simulink model "joint_test_dis_massless_2GBlks1"  (R2016b)
settings: Solver=VariableStepAuto  StartTime=0.0  StopTime=10.0  RelTol=1e-3
libraries: sm_lib x10
settings Model: Creator=smiller  LastModifiedBy=smiller

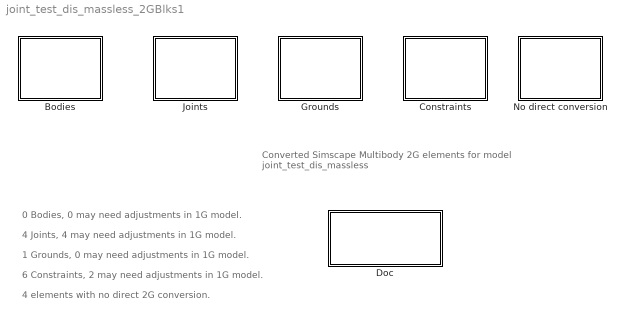
== system joint_test_dis_massless_2GBlks1 ==
  note: Converted Simscape Multibody 2G elements for model
      | joint_test_dis_massless
  note: 0 Bodies, 0 may need adjustments in 1G model.
  note: 4 Joints, 4 may need adjustments in 1G model.
  note: 1 Grounds, 0 may need adjustments in 1G model.
  note: 6 Constraints, 2 may need adjustments in 1G model.
  note: 4 elements with no direct 2G conversion.
  Bodies : Subsystem
  Constraints : Subsystem
  Doc : Subsystem
      settings: OpenFcn=web('SM1G2G_Warnings_Help.html');
      mask Display: disp('Double-click\nfor Information\nabout Diagnostics');
  Grounds : Subsystem
  Joints : Subsystem
  No direct conversion : Subsystem

== system joint_test_dis_massless_2GBlks1/Bodies ==

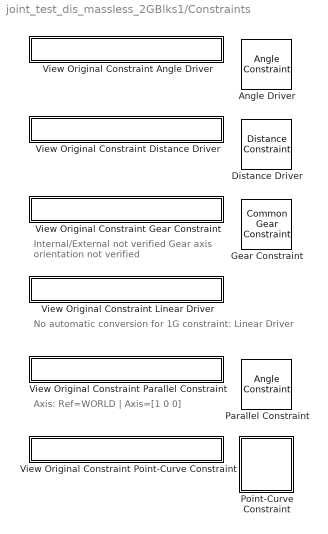
== system joint_test_dis_massless_2GBlks1/Constraints ==
  note: Internal/External not verified
      | Gear axis orientation not verified
  note: No automatic conversion for 1G constraint: Linear Driver
  note: Axis: Ref=WORLD | Axis=[1 0 0]
  Angle Driver : sm_lib/Constraints/Angle Constraint  ConstraintType=General  Angle=45  AngleUnits=deg  SenseSignedTorqueMagnitude=off  SenseTorque=off  SenseForce=off  WrenchDir=FollowerOnBase  WrenchFrame=BaseFrame
  Distance Driver : sm_lib/Constraints/Distance Constraint  Distance=1  DistanceUnits=m  SenseSignedForceMagnitude=off  SenseTorque=off  SenseForce=off  WrenchDir=FollowerOnBase  WrenchFrame=BaseFrame
  Gear Constraint : sm_lib/Gears and Couplings/Gears/Common Gear Constraint  GearType=External  SpecificationType=PitchCircleRadii  CenterDistance=20.0  CenterDistanceUnits=cm  GearRatio=1.0  BaseGearRadius=1  BaseGearRadiusUnits=m  FollGearRadius=1  FollGearRadiusUnits=m  AssemblyGearRotation=Free
  Parallel Constraint : sm_lib/Constraints/Angle Constraint  ConstraintType=Parallel  Angle=45  AngleUnits=deg  SenseSignedTorqueMagnitude=off  SenseTorque=off  SenseForce=off  WrenchDir=FollowerOnBase  WrenchFrame=BaseFrame
  Point-Curve Constraint : Subsystem
  View Original Constraint Angle Driver : Subsystem
      settings: OpenFcn=hilite_system('joint_test_dis_massless/Angle Driver');
      mask Display: disp(['View Original Constraint Angle Driver']);
  View Original Constraint Distance Driver : Subsystem
      settings: OpenFcn=hilite_system('joint_test_dis_massless/Distance Driver');
      mask Display: disp(['View Original Constraint Distance Driver']);
  View Original Constraint Gear Constraint : Subsystem
      settings: OpenFcn=hilite_system('joint_test_dis_massless/Gear Constraint');
      mask Display: disp(['View Original Constraint Gear Constraint']);
  View Original Constraint Linear Driver : Subsystem
      settings: OpenFcn=hilite_system('joint_test_dis_massless/Linear Driver');
      mask Display: disp(['View Original Constraint Linear Driver']);
  View Original Constraint Parallel Constraint : Subsystem
      settings: OpenFcn=hilite_system('joint_test_dis_massless/Parallel Constraint');
      mask Display: disp(['View Original Constraint Parallel Constraint']);
  View Original Constraint Point-Curve Constraint : Subsystem
      settings: OpenFcn=hilite_system('joint_test_dis_massless/Point-Curve Constraint');
      mask Display: disp(['View Original Constraint Point-Curve Constraint']);

== system joint_test_dis_massless_2GBlks1/Doc ==

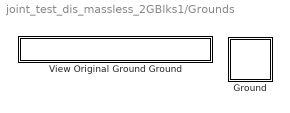
== system joint_test_dis_massless_2GBlks1/Grounds ==
  Ground : Subsystem
  View Original Ground Ground : Subsystem
      settings: OpenFcn=hilite_system('joint_test_dis_massless/Ground');
      mask Display: disp(['View Original Ground Ground']);

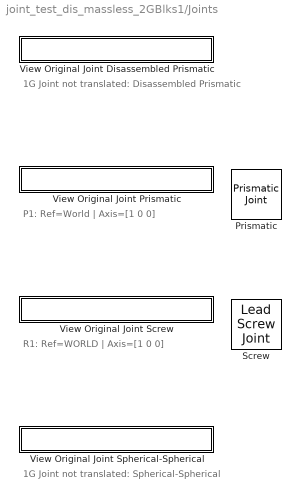
== system joint_test_dis_massless_2GBlks1/Joints ==
  note: 1G Joint not translated: Disassembled Prismatic
  note: P1: Ref=World | Axis=[1 0 0]
  note: R1: Ref=WORLD | Axis=[1 0 0]
  note: 1G Joint not translated: Spherical-Spherical
  Prismatic : sm_lib/Joints/Prismatic Joint  SenseConstraintForce=off  SenseConstraintForceX=off  SenseConstraintForceY=off  SenseConstraintForceZ=off  SenseConstraintTorque=off  SenseConstraintTorqueX=off  SenseConstraintTorqueY=off  SenseConstraintTorqueZ=off  SenseTotalForce=off  SenseTotalForceX=off  SenseTotalForceY=off  SenseTotalForceZ=off  SenseTotalTorque=off  SenseTotalTorqueX=off  SenseTotalTorqueY=off  SenseTotalTorqueZ=off  CompositeWrenchDir=FollowerOnBase  CompositeWrenchFrame=BaseFrame  EquilibriumPosition=0  EquilibriumPositionUnits=m  SpringStiffness=0  SpringStiffnessUnits=N/m  DampingCoefficient=0  DampingCoefficientUnits=N/(m/s)  TorqueActuationMode=NoTorque  MotionActuationMode=ComputedMotion  SensePosition=off  SenseVelocity=off  SenseAcceleration=off  SenseTorqueForce=off  PositionTargetSpecify=off  PositionTargetPriority=High  PositionTargetValue=0  PositionTargetValueUnits=m  VelocityTargetSpecify=off  VelocityTargetPriority=High  VelocityTargetValue=0  VelocityTargetValueUnits=m/s
  Screw : sm_lib/Joints/Lead Screw Joint  SenseConstraintForce=off  SenseConstraintForceX=off  SenseConstraintForceY=off  SenseConstraintForceZ=off  SenseConstraintTorque=off  SenseConstraintTorqueX=off  SenseConstraintTorqueY=off  SenseConstraintTorqueZ=off  SenseTotalForce=off  SenseTotalForceX=off  SenseTotalForceY=off  SenseTotalForceZ=off  SenseTotalTorque=off  SenseTotalTorqueX=off  SenseTotalTorqueY=off  SenseTotalTorqueZ=off  CompositeWrenchDir=FollowerOnBase  CompositeWrenchFrame=BaseFrame  Direction=RightHand  Lead=1  LeadUnits=mm/rev  SenseRotationPosition=off  SenseRotationVelocity=off  SenseRotationAcceleration=off  SenseTranslationPosition=off  SenseTranslationVelocity=off  SenseTranslationAcceleration=off  PositionTargetSpecify=off  PositionTargetPriority=High  PositionTargetRotationBased=off  PositionTargetRotationValue=0  PositionTargetRotationValueUnits=deg  PositionTargetTranslationValue=0  PositionTargetTranslationValueUnits=m  VelocityTargetSpecify=off  VelocityTargetPriority=High  VelocityTargetRotationBased=off  VelocityTargetRotationValue=0  VelocityTargetRotationValueUnits=deg/s  VelocityTargetTranslationValue=0  VelocityTargetTranslationValueUnits=m/s
  View Original Joint Disassembled Prismatic : Subsystem
      settings: OpenFcn=hilite_system('joint_test_dis_massless/Disassembled Prismatic');
      mask Display: disp([' View Original Joint Disassembled Prismatic']);
  View Original Joint Prismatic : Subsystem
      settings: OpenFcn=hilite_system('joint_test_dis_massless/Prismatic');
      mask Display: disp([' View Original Joint Prismatic']);
  View Original Joint Screw : Subsystem
      settings: OpenFcn=hilite_system('joint_test_dis_massless/Screw');
      mask Display: disp([' View Original Joint Screw']);
  View Original Joint Spherical-Spherical : Subsystem
      settings: OpenFcn=hilite_system('joint_test_dis_massless/Spherical-Spherical');
      mask Display: disp([' View Original Joint Spherical-Spherical']);

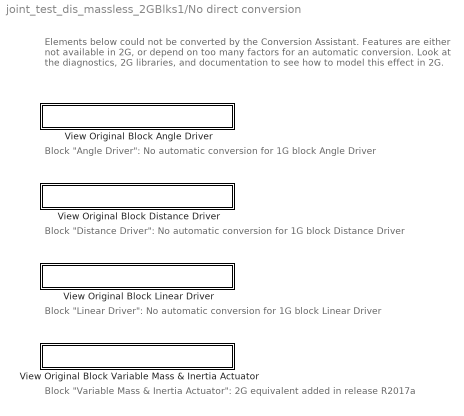
== system joint_test_dis_massless_2GBlks1/No direct conversion ==
  note: Block "Angle Driver": No automatic conversion for 1G block Angle Driver
  note: Block "Distance Driver": No automatic conversion for 1G block Distance Driver
  note: Block "Linear Driver": No automatic conversion for 1G block Linear Driver
  note: Block "Variable Mass & Inertia Actuator": 2G equivalent added in release R2017a
  note: Elements below could not be converted by the Conversion Assistant.
      | Features are either not available in 2G, or depend on too many factors
      | for an automatic conversion. Look at the diagnostics, 2G libraries, and
      | documentation to see how to model this effect in 2G.
  View Original Block Angle Driver : Subsystem
      settings: OpenFcn=hilite_system('joint_test_dis_massless/Angle Driver');
      mask Display: disp([' View Original Block Angle Driver']);
  View Original Block Distance Driver : Subsystem
      settings: OpenFcn=hilite_system('joint_test_dis_massless/Distance Driver');
      mask Display: disp([' View Original Block Distance Driver']);
  View Original Block Linear Driver : Subsystem
      settings: OpenFcn=hilite_system('joint_test_dis_massless/Linear Driver');
      mask Display: disp([' View Original Block Linear Driver']);
  View Original Block Variable Mass & Inertia Actuator : Subsystem
      settings: OpenFcn=hilite_system('joint_test_dis_massless/Variable Mass & Inertia Actuator');
      mask Display: disp([' View Original Block Variable Mass & Inertia Actuator']);

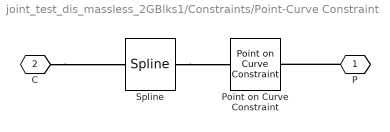
== system joint_test_dis_massless_2GBlks1/Constraints/Point-Curve Constraint ==
  Point on Curve Constraint : sm_lib/Constraints/Point on Curve Constraint  SenseTorque=off  SenseForce=off  WrenchDir=FollowerOnBase  WrenchFrame=BaseFrame
  Spline : sm_lib/Curves and Surfaces/Spline  DataPoints="[reshape([1     0.77547    0.058989    -0.52528    -0.55899    -0.17022     0.65485],[],1) reshape([0     0.42955     0.56832     0.29503    -0.12733    -0.36512    -0.39199],[],1) reshape([-0.0031056     0.36957     0.56832     0.29503    -0.12733    -0.46273    -0.40062]*0,[],1)]"  DataPointsUnits=m  EndConditionType=Closed  GraphicType=FromGeometry  MarkerShape=Sphere  MarkerSize=10  GraphicVisPropType=SimpleVisualProperties  GraphicDiffuseColor=[0 0 0]  GraphicSpecularColor=[0.5 0.5 0.5 1.0]  GraphicAmbientColor=[0.15 0.15 0.15 1.0]  GraphicEmissiveColor=[0.0 0.0 0.0 1.0]  GraphicShininess=75  GraphicOpacity=1.0
  P : PMIOPort  Port=1  Side=Left
  C : PMIOPort  Port=2  Side=Right
  connections:
  Spline/RConn1 -- Point on Curve Constraint/LConn1
  P/RConn1 -- Point on Curve Constraint/RConn1
  C/RConn1 -- Spline/LConn1

== system joint_test_dis_massless_2GBlks1/Constraints/View Original Constraint Angle Driver ==

== system joint_test_dis_massless_2GBlks1/Constraints/View Original Constraint Distance Driver ==

== system joint_test_dis_massless_2GBlks1/Constraints/View Original Constraint Gear Constraint ==

== system joint_test_dis_massless_2GBlks1/Constraints/View Original Constraint Linear Driver ==

== system joint_test_dis_massless_2GBlks1/Constraints/View Original Constraint Parallel Constraint ==

== system joint_test_dis_massless_2GBlks1/Constraints/View Original Constraint Point-Curve Constraint ==

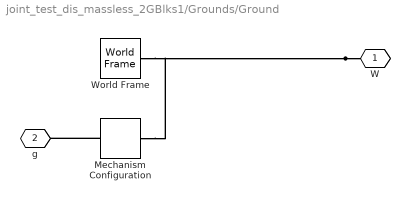
== system joint_test_dis_massless_2GBlks1/Grounds/Ground ==
  Mechanism Configuration : sm_lib/Utilities/Mechanism Configuration  UniformGravity=TimeVarying  GravityVector=[0 -9.81 0]  GravityUnits=m/s^2  LinearizationDelta=0.001
  World Frame : sm_lib/Frames and Transforms/World Frame
  W : PMIOPort  Port=1  Side=Right
  g : PMIOPort  Port=2  Side=Left
  connections:
  W/RConn1 -- World Frame/RConn1 -- Mechanism Configuration/RConn1
  Mechanism Configuration/LConn1 -- g/RConn1

== system joint_test_dis_massless_2GBlks1/Grounds/View Original Ground Ground ==

== system joint_test_dis_massless_2GBlks1/Joints/View Original Joint Disassembled Prismatic ==

== system joint_test_dis_massless_2GBlks1/Joints/View Original Joint Prismatic ==

== system joint_test_dis_massless_2GBlks1/Joints/View Original Joint Screw ==

== system joint_test_dis_massless_2GBlks1/Joints/View Original Joint Spherical-Spherical ==

== system joint_test_dis_massless_2GBlks1/No direct conversion/View Original Block Angle Driver ==

== system joint_test_dis_massless_2GBlks1/No direct conversion/View Original Block Distance Driver ==

== system joint_test_dis_massless_2GBlks1/No direct conversion/View Original Block Linear Driver ==

== system joint_test_dis_massless_2GBlks1/No direct conversion/View Original Block Variable Mass & Inertia Actuator ==
